simulink library "sm_trackV_lib_terrain_contact_elem"  (R2026a)
settings: Solver=VariableStepAuto
undefined symbols (not defined in the file): Scene
libraries: sm_rollerV_lib_terrain_contact_belem x2, sm_lib x2
Description:
  | Copyright 2024-2026 The MathWorks, Inc.
settings Model: Creator=smiller  LastModifiedBy=smiller

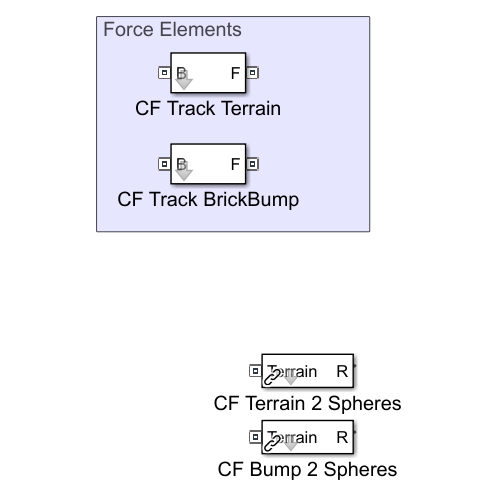
[thumbnail: Simulink's stored preview of the top-level diagram]
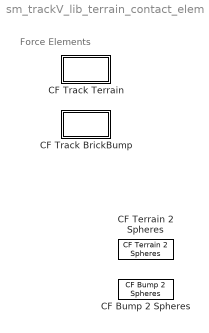
== system sm_trackV_lib_terrain_contact_elem ==
  note: Force Elements
  CF Bump 2 Spheres : sm_rollerV_lib_terrain_contact_belem/CF Bump 2 Spheres  K_BrickBump=Scene.Contact.BrickBump.K  B_BrickBump=Scene.Contact.BrickBump.B  TW_BrickBump=Scene.Contact.BrickBump.TW  CoefficientOfDynamicFriction=Scene.Contact.Terrain.mud  CoefficientOfStaticFriction=Scene.Contact.Terrain.mus  FrictionalCriticalVelocity=Scene.Contact.Terrain.CV
  CF Terrain 2 Spheres : sm_rollerV_lib_terrain_contact_belem/CF Terrain 2 Spheres  NormalStiffness=Scene.Contact.Spheres.Terrain.K  NormalDamping=Scene.Contact.Spheres.Terrain.B  NormalTransitionRegionWidth=Scene.Contact.Spheres.Terrain.TW  CoefficientOfDynamicFriction=Scene.Contact.Spheres.Terrain.mud  CoefficientOfStaticFriction=Scene.Contact.Spheres.Terrain.mus  FrictionalCriticalVelocity=Scene.Contact.Spheres.Terrain.CV
  CF Track BrickBump : Subsystem  mask(Contact Force, Track Segment to Bump){NormalStiffness=Scene.Contact.BrickBump.K, NormalDamping=Scene.Contact.BrickBump.B, NormalTransitionRegionWidth=Scene.Contact.BrickBump.TW}
      mask prompts: NormalStiffness "Normal Stiffness (N/m)"; NormalDamping "Normal Damping (N/(m/s))"; NormalTransitionRegionWidth "Normal Transition Width (m)"
      mask help: Models contact force between a track segment and a bump.
      mask TypeOptions NormalStiffness:
      | Spatial
      | Contact Force/NormalStiffness
      mask TypeOptions NormalDamping:
      | Spatial
      | Contact Force/NormalDamping
      mask TypeOptions NormalTransitionRegionWidth:
      | Spatial
      | Contact Force/NormalTransitionRegionWidth
  CF Track Terrain : Subsystem  mask(Contact Force, Track Segment to Terrain){NormalStiffness=Scene.Contact.Terrain.K, NormalDamping=Scene.Contact.Terrain.B, NormalTransitionRegionWidth=Scene.Contact.Terrain.TW, CoefficientOfDynamicFriction=Scene.Contact.Terrain.mud, CoefficientOfStaticFriction=Scene.Contact.Terrain.mus, FrictionalCriticalVelocity=Scene.Contact.Terrain.CV}
      mask prompts: NormalStiffness "Normal Stiffness (N/m)"; NormalDamping "Normal Damping (N/(m/s))"; NormalTransitionRegionWidth "Normal Transition Width (m)"; CoefficientOfDynamicFriction "Coefficient of Dynamic Friction"; CoefficientOfStaticFriction "Coefficient of Static Friction"; FrictionalCriticalVelocity "Critical Velocity (m/s)"
      mask help: Models contact force between one track segment and the terrain.
      mask TypeOptions NormalStiffness:
      | Spatial
      | Contact Force/NormalStiffness
      mask TypeOptions NormalDamping:
      | Spatial
      | Contact Force/NormalDamping
      mask TypeOptions NormalTransitionRegionWidth:
      | Spatial
      | Contact Force/NormalTransitionRegionWidth
      mask TypeOptions CoefficientOfDynamicFriction:
      | Spatial
      | Contact Force/CoefficientOfDynamicFriction
      mask TypeOptions CoefficientOfStaticFriction:
      | Spatial
      | Contact Force/CoefficientOfStaticFriction
      mask TypeOptions FrictionalCriticalVelocity:
      | Spatial
      | Contact Force/FrictionalCriticalVelocity

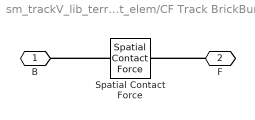
== system sm_trackV_lib_terrain_contact_elem/CF Track BrickBump ==
  Spatial Contact Force : sm_lib/Forces and Torques/Spatial Contact Force  SenseSeparationDistance=off  NormalForceType=SmoothSpringDamper  NormalStiffness=NormalStiffness  NormalStiffnessUnits=N/m  NormalDamping=NormalDamping  NormalDampingUnits=N/(m/s)  NormalTransitionRegionWidth=NormalTransitionRegionWidth  NormalTransitionRegionWidthUnits=m  FrictionType=None  CoefficientOfStaticFriction=0.5  CoefficientOfDynamicFriction=0.5  FrictionalCriticalVelocity=1e-3  FrictionalCriticalVelocityUnits=m/s  SenseContactSignal=off  SensePenetrationDepth=off  SenseNormalVelocity=off  SenseTangentialVelocity=off  SensingForceTorqueDirection=BaseOnFollower  SensingForceTorqueResolutionFrame=ContactFrame  SenseNormalForce=off  SenseNormalForceMagnitude=off  SenseNormalTorque=off  SenseFrictionalForce=off  SenseFrictionalForceMagnitude=off  SenseFrictionalTorque=off  SenseTotalForce=off  SenseTotalTorque=off  SenseContactBaseRotation=off  SenseContactBaseTranslation=off  SenseContactFollowerRotation=off  SenseContactFollowerTranslation=off  ZeroCrossDetectContactStartAndEnd=off
  B : PMIOPort  Side=Left
  F : PMIOPort  Port=2  Side=Right
  connections:
  F/RConn1 -- Spatial Contact Force/RConn1
  Spatial Contact Force/LConn1 -- B/RConn1

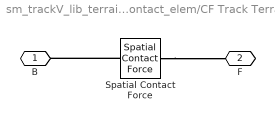
== system sm_trackV_lib_terrain_contact_elem/CF Track Terrain ==
  Spatial Contact Force : sm_lib/Forces and Torques/Spatial Contact Force  SenseSeparationDistance=off  NormalForceType=SmoothSpringDamper  NormalStiffness=NormalStiffness  NormalStiffnessUnits=N/m  NormalDamping=NormalDamping  NormalDampingUnits=N/(m/s)  NormalTransitionRegionWidth=NormalTransitionRegionWidth  NormalTransitionRegionWidthUnits=m  FrictionType=SmoothStickSlip  CoefficientOfStaticFriction=CoefficientOfStaticFriction  CoefficientOfDynamicFriction=CoefficientOfDynamicFriction  FrictionalCriticalVelocity=FrictionalCriticalVelocity  FrictionalCriticalVelocityUnits=m/s  SenseContactSignal=off  SensePenetrationDepth=off  SenseNormalVelocity=off  SenseTangentialVelocity=off  SensingForceTorqueDirection=BaseOnFollower  SensingForceTorqueResolutionFrame=ContactFrame  SenseNormalForce=off  SenseNormalForceMagnitude=off  SenseNormalTorque=off  SenseFrictionalForce=off  SenseFrictionalForceMagnitude=off  SenseFrictionalTorque=off  SenseTotalForce=off  SenseTotalTorque=off  SenseContactBaseRotation=off  SenseContactBaseTranslation=off  SenseContactFollowerRotation=off  SenseContactFollowerTranslation=off  ZeroCrossDetectContactStartAndEnd=off
  B : PMIOPort  Side=Left
  F : PMIOPort  Port=2  Side=Right
  connections:
  Spatial Contact Force/LConn1 -- B/RConn1
  Spatial Contact Force/RConn1 -- F/RConn1
